simulink model "TorqueVect"  (Simulink 10.1)
settings: Solver=ode45  StartTime=0.0  StopTime=inf  RelTol=1e-3  EnableMultiTasking=on
PreLoadFcn:
  | run('Parameters\FSE_Parameters.m')
undefined symbols (not defined in the file): TC_Decr_Gas, TC_Derivative, TC_Incr_Gas, TC_On, TC_Relay_Off, TC_Relay_On, TV_On, TV_Override
libraries: CarMaker4SL x33, simulink x5, simulink_extras x4
(part 2 of 3)

== system TorqueVect/CarMaker/IPG Vehicle/CarAndTrailer/Forces/Tires ==
  note: The TireXX_Out signals will only be used if FileIdent is "CarMaker-Tire-CM4SL" in the tire parameter file!
      | An example parameter file can be found in Data/Tire/DT_CM4SL_UserTire.
  Sync_In : Inport
  TireFL_In : Inport  Port=2
  TireFR_In : Inport  Port=3
  TireRL_In : Inport  Port=4
  TireRR_In : Inport  Port=5
  Bus Creator{1..4} (4 alike) : BusCreator  Inputs=11
  Demux{1..3,8} (4 alike) : Demux  Outputs=7
      settings: DisplayOption=none
  TireFL : Subsystem
  TireFR : Subsystem
  TireRL : Subsystem
  TireRR : Subsystem
  TireFL_Out : Outport
  TireFR_Out : Outport  Port=2
  TireRL_Out : Outport  Port=3
  TireRR_Out : Outport  Port=4
  wires:
  Sync_In/1 -> TireRR/1(Sync_In), TireRL/1(Sync_In), TireFR/1(Sync_In), TireFL/1(Sync_In)
  Bus Creator4/1 -> TireRR_Out/1
  Bus Creator2/1 -> TireRL_Out/1
  Bus Creator1/1 -> TireFR_Out/1
  Demux3/5 -> TireRR/6(Rim_turnv)  "Tire_In Rim_turnv"
  Demux3/4 -> TireRR/5(Rim_rotv)  "Tire_In Rim_rotv"
  Demux3/1 -> TireRR/2(Load)  "Tire_In Load"
  Demux3/7 -> TireRR/8(muRoad)  "Tire_In mu"
  Demux3/6 -> TireRR/7(InclinAngle)  "Tire_In Camber"
  Demux3/2 -> TireRR/3(vxtrans)  "Tire_In vxtrans"
  Demux3/3 -> TireRR/4(vytrans)  "Tire_In vytrans"
  TireRR/11(AlignTrq) -> Bus Creator4/11  "Tire_Out AlignTrq"
  TireRR/10(RollResist) -> Bus Creator4/10  "Tire_Out RollResist"
  TireRR/9(OverturnTrq) -> Bus Creator4/9  "Tire_Out OverturnTrq"
  TireRR/8(LoadFrc) -> Bus Creator4/8  "Tire_Out LoadFrc"
  TireRR/7(SideFrc) -> Bus Creator4/7  "Tire_Out SideFrc"
  TireRR/6(LongFrc) -> Bus Creator4/6  "Tire_Out LongFrc"
  TireRR/5(vBelt) -> Bus Creator4/5  "Tire_Out vBelt"
  TireRR/4(rBelt_eff) -> Bus Creator4/4  "Tire_Out rBelt_eff"
  TireRR/3(TurnSlp) -> Bus Creator4/3  "Tire_Out TurnSlp"
  TireRR/1(Slp) -> Bus Creator4/1  "Tire_Out Slp"
  TireRR/2(Alpha) -> Bus Creator4/2  "Tire_Out Alpha"
  Demux2/5 -> TireRL/6(Rim_turnv)  "Tire_In Rim_turnv"
  Demux2/4 -> TireRL/5(Rim_rotv)  "Tire_In Rim_rotv"
  Demux2/1 -> TireRL/2(Load)  "Tire_In Load"
  Demux2/7 -> TireRL/8(muRoad)  "Tire_In mu"
  Demux2/6 -> TireRL/7(InclinAngle)  "Tire_In Camber"
  Demux2/2 -> TireRL/3(vxtrans)  "Tire_In vxtrans"
  Demux2/3 -> TireRL/4(vytrans)  "Tire_In vytrans"
  TireRL/11(AlignTrq) -> Bus Creator2/11  "Tire_Out AlignTrq"
  TireRL/10(RollResist) -> Bus Creator2/10  "Tire_Out RollResist"
  TireRL/9(OverturnTrq) -> Bus Creator2/9  "Tire_Out OverturnTrq"
  TireRL/8(LoadFrc) -> Bus Creator2/8  "Tire_Out LoadFrc"
  TireRL/7(SideFrc) -> Bus Creator2/7  "Tire_Out SideFrc"
  TireRL/6(LongFrc) -> Bus Creator2/6  "Tire_Out LongFrc"
  TireRL/5(vBelt) -> Bus Creator2/5  "Tire_Out vBelt"
  TireRL/4(rBelt_eff) -> Bus Creator2/4  "Tire_Out rBelt_eff"
  TireRL/3(TurnSlp) -> Bus Creator2/3  "Tire_Out TurnSlp"
  TireRL/1(Slp) -> Bus Creator2/1  "Tire_Out Slp"
  TireRL/2(Alpha) -> Bus Creator2/2  "Tire_Out Alpha"
  Demux1/5 -> TireFR/6(Rim_turnv)  "Tire_In Rim_turnv"
  Demux1/4 -> TireFR/5(Rim_rotv)  "Tire_In Rim_rotv"
  Demux1/1 -> TireFR/2(Load)  "Tire_In Load"
  Demux1/7 -> TireFR/8(muRoad)  "Tire_In mu"
  Demux1/6 -> TireFR/7(InclinAngle)  "Tire_In Camber"
  Demux1/2 -> TireFR/3(vxtrans)  "Tire_In vxtrans"
  Demux1/3 -> TireFR/4(vytrans)  "Tire_In vytrans"
  TireFR/11(AlignTrq) -> Bus Creator1/11  "Tire_Out AlignTrq"
  TireFR/10(RollResist) -> Bus Creator1/10  "Tire_Out RollResist"
  TireFR/9(OverturnTrq) -> Bus Creator1/9  "Tire_Out OverturnTrq"
  TireFR/8(LoadFrc) -> Bus Creator1/8  "Tire_Out LoadFrc"
  TireFR/7(SideFrc) -> Bus Creator1/7  "Tire_Out SideFrc"
  TireFR/6(LongFrc) -> Bus Creator1/6  "Tire_Out LongFrc"
  TireFR/5(vBelt) -> Bus Creator1/5  "Tire_Out vBelt"
  TireFR/4(rBelt_eff) -> Bus Creator1/4  "Tire_Out rBelt_eff"
  TireFR/3(TurnSlp) -> Bus Creator1/3  "Tire_Out TurnSlp"
  TireFR/1(Slp) -> Bus Creator1/1  "Tire_Out Slp"
  TireFR/2(Alpha) -> Bus Creator1/2  "Tire_Out Alpha"
  Demux8/5 -> TireFL/6(Rim_turnv)  "Tire_In Rim_turnv"
  Demux8/4 -> TireFL/5(Rim_rotv)  "Tire_In Rim_rotv"
  TireFL_In/1 -> Demux8/1
  Demux8/1 -> TireFL/2(Load)  "Tire_In Load"
  Demux8/7 -> TireFL/8(muRoad)  "Tire_In mu"
  Demux8/6 -> TireFL/7(InclinAngle)  "Tire_In Camber"
  Demux8/2 -> TireFL/3(vxtrans)  "Tire_In vxtrans"
  Demux8/3 -> TireFL/4(vytrans)  "Tire_In vytrans"
  TireFL/11(AlignTrq) -> Bus Creator3/11  "Tire_Out AlignTrq"
  TireFL/10(RollResist) -> Bus Creator3/10  "Tire_Out RollResist"
  TireFL/9(OverturnTrq) -> Bus Creator3/9  "Tire_Out OverturnTrq"
  TireFL/8(LoadFrc) -> Bus Creator3/8  "Tire_Out LoadFrc"
  TireFL/7(SideFrc) -> Bus Creator3/7  "Tire_Out SideFrc"
  TireFL/6(LongFrc) -> Bus Creator3/6  "Tire_Out LongFrc"
  TireFL/5(vBelt) -> Bus Creator3/5  "Tire_Out vBelt"
  TireFL/4(rBelt_eff) -> Bus Creator3/4  "Tire_Out rBelt_eff"
  TireFL/3(TurnSlp) -> Bus Creator3/3  "Tire_Out TurnSlp"
  TireFL/1(Slp) -> Bus Creator3/1  "Tire_Out Slp"
  TireFL/2(Alpha) -> Bus Creator3/2  "Tire_Out Alpha"
  Bus Creator3/1 -> TireFL_Out/1
  TireFR_In/1 -> Demux1/1
  TireRL_In/1 -> Demux2/1
  TireRR_In/1 -> Demux3/1

== system TorqueVect/CarMaker/IPG Vehicle/CarAndTrailer/Forces/Vehicle Forces ==
  Sync_In : Inport
  Bus Creator1 : BusCreator  Inputs=12
  Bus Creator8 : BusCreator  Inputs=16
  BusCreator1 : BusCreator  Inputs=4
  BusCreator2 : BusCreator  Inputs=9
  Demux : Demux  Outputs=16
      settings: DisplayOption=none
  Demux1 : Demux  Outputs=12
      settings: DisplayOption=none
  Demux2 : Demux  Outputs=13
      settings: DisplayOption=none
  Forces : S-Function  FunctionName=CM_Sfun  Parameters='Forces'  SFunctionDeploymentMode=off  EnableBusSupport=off
  Terminator : Terminator
  Sync_Out : Outport
  Car.Virtual : Outport  Port=2
  Car.Aero : Outport  Port=3
  Car.Load : Outport  Port=4
  wires:
  BusCreator1/1 -> Terminator/1  "Aero IF (in)"
  Demux2/13 -> BusCreator2/9  "car Aero Trq_1 z"
  Demux2/12 -> BusCreator2/8  "car Aero Trq_1 y"
  Demux2/11 -> BusCreator2/7  "car Aero Trq_1 x"
  Demux2/10 -> BusCreator2/6  "car Aero Frc_1 z"
  Demux2/9 -> BusCreator2/5  "car Aero Frc_1 y"
  Demux2/8 -> BusCreator2/4  "car Aero Frc_1 x"
  Demux2/7 -> BusCreator2/3  "car Aero PoA_1 z"
  Demux2/6 -> BusCreator2/2  "car Aero PoA_1 y"
  Demux2/5 -> BusCreator2/1  "car Aero PoA_1 x"
  Demux2/4 -> BusCreator1/4  "car Aero tau_1"
  Demux2/3 -> BusCreator1/3  "car Aero ApproachVel_1 z"
  Demux2/2 -> BusCreator1/2  "car Aero ApproachVel_1 y"
  Demux2/1 -> BusCreator1/1  "car Aero ApproachVel_1 x"
  Demux/16 -> Bus Creator8/16  "Car Load_3 tz"
  Demux/15 -> Bus Creator8/15  "Car Load_3 ty"
  Demux/14 -> Bus Creator8/14  "Car Load_3 tx"
  Demux/13 -> Bus Creator8/13  "Car Load_3 mass"
  Demux1/12 -> Bus Creator1/12  "Car Virtual Trq_0 z"
  Demux1/11 -> Bus Creator1/11  "Car Virtual Trq_0 y"
  Demux1/10 -> Bus Creator1/10  "Car Virtual Trq_0 x"
  Demux1/9 -> Bus Creator1/9  "Car Virtual Trq_1 z"
  Demux1/8 -> Bus Creator1/8  "Car Virtual Trq_1 y"
  Demux1/7 -> Bus Creator1/7  "Car Virtual Trq_1 x"
  Demux1/6 -> Bus Creator1/6  "Car Virtual Frc_0 z"
  Demux1/5 -> Bus Creator1/5  "Car Virtual Frc_0 y"
  Demux1/4 -> Bus Creator1/4  "Car Virtual Frc_0 x"
  Sync_In/1 -> Forces/1
  Forces/1 -> Sync_Out/1
  BusCreator2/1 -> Car.Aero/1
  Demux1/1 -> Bus Creator1/1  "Car Virtual Frc_1 x"
  Demux1/2 -> Bus Creator1/2  "Car Virtual Frc_1 y"
  Demux1/3 -> Bus Creator1/3  "Car Virtual Frc_1 z"
  Forces/3 -> Demux2/1
  Forces/2 -> Demux1/1
  Bus Creator1/1 -> Car.Virtual/1
  Bus Creator8/1 -> Car.Load/1
  Demux/1 -> Bus Creator8/1  "Car Load_0 mass"
  Demux/2 -> Bus Creator8/2  "Car Load_0 tx"
  Demux/3 -> Bus Creator8/3  "Car Load_0 ty"
  Demux/4 -> Bus Creator8/4  "Car Load_0 tz"
  Demux/5 -> Bus Creator8/5  "Car Load_1 mass"
  Demux/6 -> Bus Creator8/6  "Car Load_1 tx"
  Demux/7 -> Bus Creator8/7  "Car Load_1 ty"
  Demux/8 -> Bus Creator8/8  "Car Load_1 tz"
  Demux/9 -> Bus Creator8/9  "Car Load_2 mass"
  Demux/10 -> Bus Creator8/10  "Car Load_2 tx"
  Demux/11 -> Bus Creator8/11  "Car Load_2 ty"
  Demux/12 -> Bus Creator8/12  "Car Load_2 tz"
  Forces/4 -> Demux/1

== system TorqueVect/CarMaker/IPG Vehicle/CarAndTrailer/Trailer/CreateBus Car.Hitch.FrcTrq ==
  In1 : Inport
  Bus Creator7 : BusCreator  Inputs=6
  Demux7 : Demux  Outputs=6
      settings: DisplayOption=none
  Out1 : Outport
  wires:
  In1/1 -> Demux7/1
  Bus Creator7/1 -> Out1/1
  Demux7/6 -> Bus Creator7/6  "Car Hitch Trq2Car z"
  Demux7/5 -> Bus Creator7/5  "Car Hitch Trq2Car y"
  Demux7/4 -> Bus Creator7/4  "Car Hitch Trq2Car x"
  Demux7/3 -> Bus Creator7/3  "Car Hitch Frc2Car z"
  Demux7/2 -> Bus Creator7/2  "Car Hitch Frc2Car y"
  Demux7/1 -> Bus Creator7/1  "Car Hitch Frc2Car x"

== system TorqueVect/CarMaker/IPG Vehicle/CarAndTrailer/Trailer/CreateBus Vhcl.Motion ==
  In1 : Inport
  BusCreator : BusCreator  Inputs=15
  Demux : Demux  Outputs=15
      settings: DisplayOption=none
  Out1 : Outport
  wires:
  Demux/15 -> BusCreator/15  "Vhcl YawAcc"
  Demux/14 -> BusCreator/14  "Vhcl YawVel"
  Demux/13 -> BusCreator/13  "Vhcl Yaw"
  Demux/12 -> BusCreator/12  "Vhcl PitchAcc"
  Demux/11 -> BusCreator/11  "Vhcl PitchVel"
  Demux/10 -> BusCreator/10  "Vhcl Pitch"
  Demux/9 -> BusCreator/9  "Vhcl RollAcc"
  Demux/8 -> BusCreator/8  "Vhcl RollVel"
  Demux/7 -> BusCreator/7  "Vhcl Roll"
  Demux/6 -> BusCreator/6  "Vhcl Hitch_Pos z"
  Demux/5 -> BusCreator/5  "Vhcl Hitch_Pos y"
  Demux/4 -> BusCreator/4  "Vhcl Hitch_Pos x"
  Demux/3 -> BusCreator/3  "Vhcl sRoad"
  Demux/2 -> BusCreator/2  "Vhcl Distance"
  Demux/1 -> BusCreator/1  "Vhcl v"
  In1/1 -> Demux/1
  BusCreator/1 -> Out1/1

== system TorqueVect/CarMaker/IPG Vehicle/CarAndTrailer/Trailer/CreateBus Vhcl.PoI ==
  In1 : Inport
  Bus Creator3 : BusCreator  Inputs=18
  Demux3 : Demux  Outputs=18
      settings: DisplayOption=none
  Out1 : Outport
  wires:
  Demux3/18 -> Bus Creator3/18  "Vhcl PoI_GCS Elev"
  Demux3/17 -> Bus Creator3/17  "Vhcl PoI_GCS Lat"
  Demux3/16 -> Bus Creator3/16  "Vhcl PoI_GCS Long"
  Demux3/15 -> Bus Creator3/15  "Vhcl PoI_Acc_1 z"
  Demux3/14 -> Bus Creator3/14  "Vhcl PoI_Acc_1 y"
  Demux3/13 -> Bus Creator3/13  "Vhcl PoI_Acc_1 x"
  Demux3/12 -> Bus Creator3/12  "Vhcl PoI_Vel_1 z"
  Demux3/11 -> Bus Creator3/11  "Vhcl PoI_Vel_1 y"
  Demux3/10 -> Bus Creator3/10  "Vhcl PoI_Vel_1 x"
  Demux3/9 -> Bus Creator3/9  "Vhcl PoI_Acc z"
  Demux3/8 -> Bus Creator3/8  "Vhcl PoI_Acc y"
  Demux3/7 -> Bus Creator3/7  "Vhcl PoI_Acc x"
  Demux3/6 -> Bus Creator3/6  "Vhcl PoI_Vel z"
  Demux3/5 -> Bus Creator3/5  "Vhcl PoI_Vel y"
  Demux3/4 -> Bus Creator3/4  "Vhcl PoI_Vel x"
  Demux3/3 -> Bus Creator3/3  "Vhcl PoI_Pos z"
  Demux3/2 -> Bus Creator3/2  "Vhcl PoI_Pos y"
  In1/1 -> Demux3/1
  Bus Creator3/1 -> Out1/1
  Demux3/1 -> Bus Creator3/1  "Vhcl PoI_Pos x"

== system TorqueVect/CarMaker/IPG Vehicle/CarAndTrailer/Trailer/CreateBus Vhcl.Steering ==
  In1 : Inport
  Bus Creator3 : BusCreator  Inputs=4
  Demux : Demux
      settings: DisplayOption=none
  Out1 : Outport
  wires:
  Bus Creator3/1 -> Out1/1
  Demux/1 -> Bus Creator3/1  "Vhcl Steering Ang"
  Demux/3 -> Bus Creator3/3  "Vhcl Steering AngAcc"
  Demux/2 -> Bus Creator3/2  "Vhcl Steering AngVel"
  Demux/4 -> Bus Creator3/4  "Vhcl Steering Trq"
  In1/1 -> Demux/1

== system TorqueVect/CarMaker/IPG Vehicle/CarAndTrailer/Trailer/CreateBus Vhcl.Wheel.FL ==
  In1 : Inport
  Bus Creator3 : BusCreator  Inputs=14
  Demux3 : Demux  Outputs=14
      settings: DisplayOption=none
  Out1 : Outport
  wires:
  Demux3/14 -> Bus Creator3/14  "Vhcl Wheel FL Trq_WhlBearing"
  Demux3/13 -> Bus Creator3/13  "Vhcl Wheel FL Trq_T2W"
  Demux3/12 -> Bus Creator3/12  "Vhcl Wheel FL SideSlip"
  Demux3/11 -> Bus Creator3/11  "Vhcl Wheel FL LongSlip"
  Demux3/10 -> Bus Creator3/10  "Vhcl Wheel FL vBelt"
  Demux3/9 -> Bus Creator3/9  "Vhcl Wheel FL Fz"
  Demux3/8 -> Bus Creator3/8  "Vhcl Wheel FL Fy"
  Demux3/7 -> Bus Creator3/7  "Vhcl Wheel FL Fx"
  Demux3/6 -> Bus Creator3/6  "Vhcl Wheel FL r_zxy z"
  Demux3/5 -> Bus Creator3/5  "Vhcl Wheel FL r_zxy y"
  Demux3/4 -> Bus Creator3/4  "Vhcl Wheel FL r_zxy x"
  Demux3/3 -> Bus Creator3/3  "Vhcl Wheel FL t z"
  Demux3/2 -> Bus Creator3/2  "Vhcl Wheel FL t y"
  In1/1 -> Demux3/1
  Bus Creator3/1 -> Out1/1
  Demux3/1 -> Bus Creator3/1  "Vhcl Wheel FL t x"

== system TorqueVect/CarMaker/IPG Vehicle/CarAndTrailer/Trailer/CreateBus Vhcl.Wheel.FR ==
  In1 : Inport
  Bus Creator3 : BusCreator  Inputs=14
  Demux3 : Demux  Outputs=14
      settings: DisplayOption=none
  Out1 : Outport
  wires:
  Demux3/14 -> Bus Creator3/14  "Vhcl Wheel FR Trq_WhlBearing"
  Demux3/13 -> Bus Creator3/13  "Vhcl Wheel FR Trq_T2W"
  Demux3/12 -> Bus Creator3/12  "Vhcl Wheel FR SideSlip"
  Demux3/11 -> Bus Creator3/11  "Vhcl Wheel FR LongSlip"
  Demux3/10 -> Bus Creator3/10  "Vhcl Wheel FR vBelt"
  Demux3/9 -> Bus Creator3/9  "Vhcl Wheel FR Fz"
  Demux3/8 -> Bus Creator3/8  "Vhcl Wheel FR Fy"
  Demux3/7 -> Bus Creator3/7  "Vhcl Wheel FR Fx"
  Demux3/6 -> Bus Creator3/6  "Vhcl Wheel FR r_zxy z"
  Demux3/5 -> Bus Creator3/5  "Vhcl Wheel FR r_zxy y"
  Demux3/4 -> Bus Creator3/4  "Vhcl Wheel FR r_zxy x"
  Demux3/3 -> Bus Creator3/3  "Vhcl Wheel FR t z"
  Demux3/2 -> Bus Creator3/2  "Vhcl Wheel FR t y"
  In1/1 -> Demux3/1
  Bus Creator3/1 -> Out1/1
  Demux3/1 -> Bus Creator3/1  "Vhcl Wheel FR t x"

== system TorqueVect/CarMaker/IPG Vehicle/CarAndTrailer/Trailer/CreateBus Vhcl.Wheel.RL ==
  In1 : Inport
  Bus Creator3 : BusCreator  Inputs=14
  Demux3 : Demux  Outputs=14
      settings: DisplayOption=none
  Out1 : Outport
  wires:
  Demux3/14 -> Bus Creator3/14  "Vhcl Wheel RL Trq_WhlBearing"
  Demux3/13 -> Bus Creator3/13  "Vhcl Wheel RL Trq_T2W"
  Demux3/12 -> Bus Creator3/12  "Vhcl Wheel RL SideSlip"
  Demux3/11 -> Bus Creator3/11  "Vhcl Wheel RL LongSlip"
  Demux3/10 -> Bus Creator3/10  "Vhcl Wheel RL vBelt"
  Demux3/9 -> Bus Creator3/9  "Vhcl Wheel RL Fz"
  Demux3/8 -> Bus Creator3/8  "Vhcl Wheel RL Fy"
  Demux3/7 -> Bus Creator3/7  "Vhcl Wheel RL Fx"
  Demux3/6 -> Bus Creator3/6  "Vhcl Wheel RL r_zxy z"
  Demux3/5 -> Bus Creator3/5  "Vhcl Wheel RL r_zxy y"
  Demux3/4 -> Bus Creator3/4  "Vhcl Wheel RL r_zxy x"
  Demux3/3 -> Bus Creator3/3  "Vhcl Wheel RL t z"
  Demux3/2 -> Bus Creator3/2  "Vhcl Wheel RL t y"
  In1/1 -> Demux3/1
  Bus Creator3/1 -> Out1/1
  Demux3/1 -> Bus Creator3/1  "Vhcl Wheel RL t x"

== system TorqueVect/CarMaker/IPG Vehicle/CarAndTrailer/Trailer/CreateBus Vhcl.Wheel.RR ==
  In1 : Inport
  Bus Creator3 : BusCreator  Inputs=14
  Demux3 : Demux  Outputs=14
      settings: DisplayOption=none
  Out1 : Outport
  wires:
  Demux3/14 -> Bus Creator3/14  "Vhcl Wheel RR Trq_WhlBearing"
  Demux3/13 -> Bus Creator3/13  "Vhcl Wheel RR Trq_T2W"
  Demux3/12 -> Bus Creator3/12  "Vhcl Wheel RR SideSlip"
  Demux3/11 -> Bus Creator3/11  "Vhcl Wheel RR LongSlip"
  Demux3/10 -> Bus Creator3/10  "Vhcl Wheel RR vBelt"
  Demux3/9 -> Bus Creator3/9  "Vhcl Wheel RR Fz"
  Demux3/8 -> Bus Creator3/8  "Vhcl Wheel RR Fy"
  Demux3/7 -> Bus Creator3/7  "Vhcl Wheel RR Fx"
  Demux3/6 -> Bus Creator3/6  "Vhcl Wheel RR r_zxy z"
  Demux3/5 -> Bus Creator3/5  "Vhcl Wheel RR r_zxy y"
  Demux3/4 -> Bus Creator3/4  "Vhcl Wheel RR r_zxy x"
  Demux3/3 -> Bus Creator3/3  "Vhcl Wheel RR t z"
  Demux3/2 -> Bus Creator3/2  "Vhcl Wheel RR t y"
  In1/1 -> Demux3/1
  Bus Creator3/1 -> Out1/1
  Demux3/1 -> Bus Creator3/1  "Vhcl Wheel RR t x"

== system TorqueVect/CarMaker/IPG Vehicle/PowerTrain/PTControl Example/CreateBus PTC ClutchOut ==
  In : Inport
  BusCreator : BusCreator  Inputs=3
  Demux : Demux  Outputs=3
      settings: DisplayOption=none
  Out : Outport  VectorParamsAs1DForOutWhenUnconnected=off
  wires:
  In/1 -> Demux/1
  BusCreator/1 -> Out/1
  Demux/1 -> BusCreator/1  "PTC ClutchOut Pos"
  Demux/2 -> BusCreator/2  "PTC ClutchOut rotv_out_trg"
  Demux/3 -> BusCreator/3  "PTC ClutchOut Trq_out_trg"

== system TorqueVect/CarMaker/IPG Vehicle/PowerTrain/PTControl Example/CreateBus PTC EngineOut ==
  In : Inport
  BusCreator : BusCreator  Inputs=5
  Demux : Demux  Outputs=5
      settings: DisplayOption=none
  Out : Outport  VectorParamsAs1DForOutWhenUnconnected=off
  wires:
  In/1 -> Demux/1
  BusCreator/1 -> Out/1
  Demux/1 -> BusCreator/1  "PTC EngineOut set_ISC"
  Demux/2 -> BusCreator/2  "PTC EngineOut FuelCutOff"
  Demux/3 -> BusCreator/3  "PTC EngineOut Load"
  Demux/4 -> BusCreator/4  "PTC EngineOut Trq_trg"
  Demux/5 -> BusCreator/5  "PTC EngineOut rotv_trg"

== system TorqueVect/CarMaker/IPG Vehicle/PowerTrain/PTControl Example/CreateBus PTC GearBoxM_Out0 ==
  In : Inport
  BusCreator : BusCreator  Inputs=12
  Demux : Demux  Outputs=12
      settings: DisplayOption=none
  Out : Outport  VectorParamsAs1DForOutWhenUnconnected=off
  wires:
  In/1 -> Demux/1
  BusCreator/1 -> Out/1
  Demux/1 -> BusCreator/1  "PTC GearBoxM_Out0 GearNoTrg"
  Demux/2 -> BusCreator/2  "PTC GearBoxM_Out0 GearNoTrg_dis"
  Demux/3 -> BusCreator/3  "PTC GearBoxM_Out0 set_ParkBrake"
  Demux/4 -> BusCreator/4  "PTC GearBoxM_Out0 i_trg"
  Demux/5 -> BusCreator/5  "PTC GearBoxM_Out0 rotv_in_trg"
  Demux/6 -> BusCreator/6  "PTC GearBoxM_Out0 Trq_out_trg"
  Demux/7 -> BusCreator/7  "PTC GearBoxM_Out0 Clutch Pos"
  Demux/8 -> BusCreator/8  "PTC GearBoxM_Out0 Clutch rotv_out_trg"
  Demux/9 -> BusCreator/9  "PTC GearBoxM_Out0 Clutch Trq_out_trg"
  Demux/10 -> BusCreator/10  "PTC GearBoxM_Out0 Clutch_dis Pos"
  Demux/11 -> BusCreator/11  "PTC GearBoxM_Out0 Clutch_dis rotv_out_trg"
  Demux/12 -> BusCreator/12  "PTC GearBoxM_Out0 Clutch_dis Trq_out_trg"

== system TorqueVect/CarMaker/IPG Vehicle/PowerTrain/PTControl Example/CreateBus PTC GearBoxM_Out1 ==
  In : Inport
  BusCreator : BusCreator  Inputs=12
  Demux : Demux  Outputs=12
      settings: DisplayOption=none
  Out : Outport  VectorParamsAs1DForOutWhenUnconnected=off
  wires:
  In/1 -> Demux/1
  BusCreator/1 -> Out/1
  Demux/1 -> BusCreator/1  "PTC GearBoxM_Out1 GearNoTrg"
  Demux/2 -> BusCreator/2  "PTC GearBoxM_Out1 GearNoTrg_dis"
  Demux/3 -> BusCreator/3  "PTC GearBoxM_Out1 set_ParkBrake"
  Demux/4 -> BusCreator/4  "PTC GearBoxM_Out1 i_trg"
  Demux/5 -> BusCreator/5  "PTC GearBoxM_Out1 rotv_in_trg"
  Demux/6 -> BusCreator/6  "PTC GearBoxM_Out1 Trq_out_trg"
  Demux/7 -> BusCreator/7  "PTC GearBoxM_Out1 Clutch Pos"
  Demux/8 -> BusCreator/8  "PTC GearBoxM_Out1 Clutch rotv_out_trg"
  Demux/9 -> BusCreator/9  "PTC GearBoxM_Out1 Clutch Trq_out_trg"
  Demux/10 -> BusCreator/10  "PTC GearBoxM_Out1 Clutch_dis Pos"
  Demux/11 -> BusCreator/11  "PTC GearBoxM_Out1 Clutch_dis rotv_out_trg"
  Demux/12 -> BusCreator/12  "PTC GearBoxM_Out1 Clutch_dis Trq_out_trg"

== system TorqueVect/CarMaker/IPG Vehicle/PowerTrain/PTControl Example/CreateBus PTC GearBoxM_Out2 ==
  In : Inport
  BusCreator : BusCreator  Inputs=12
  Demux : Demux  Outputs=12
      settings: DisplayOption=none
  Out : Outport  VectorParamsAs1DForOutWhenUnconnected=off
  wires:
  In/1 -> Demux/1
  BusCreator/1 -> Out/1
  Demux/1 -> BusCreator/1  "PTC GearBoxM_Out2 GearNoTrg"
  Demux/2 -> BusCreator/2  "PTC GearBoxM_Out2 GearNoTrg_dis"
  Demux/3 -> BusCreator/3  "PTC GearBoxM_Out2 set_ParkBrake"
  Demux/4 -> BusCreator/4  "PTC GearBoxM_Out2 i_trg"
  Demux/5 -> BusCreator/5  "PTC GearBoxM_Out2 rotv_in_trg"
  Demux/6 -> BusCreator/6  "PTC GearBoxM_Out2 Trq_out_trg"
  Demux/7 -> BusCreator/7  "PTC GearBoxM_Out2 Clutch Pos"
  Demux/8 -> BusCreator/8  "PTC GearBoxM_Out2 Clutch rotv_out_trg"
  Demux/9 -> BusCreator/9  "PTC GearBoxM_Out2 Clutch Trq_out_trg"
  Demux/10 -> BusCreator/10  "PTC GearBoxM_Out2 Clutch_dis Pos"
  Demux/11 -> BusCreator/11  "PTC GearBoxM_Out2 Clutch_dis rotv_out_trg"
  Demux/12 -> BusCreator/12  "PTC GearBoxM_Out2 Clutch_dis Trq_out_trg"

== system TorqueVect/CarMaker/IPG Vehicle/PowerTrain/PTControl Example/CreateBus PTC GearBoxM_Out3 ==
  In : Inport
  BusCreator : BusCreator  Inputs=12
  Demux : Demux  Outputs=12
      settings: DisplayOption=none
  Out : Outport  VectorParamsAs1DForOutWhenUnconnected=off
  wires:
  In/1 -> Demux/1
  BusCreator/1 -> Out/1
  Demux/1 -> BusCreator/1  "PTC GearBoxM_Out3 GearNoTrg"
  Demux/2 -> BusCreator/2  "PTC GearBoxM_Out3 GearNoTrg_dis"
  Demux/3 -> BusCreator/3  "PTC GearBoxM_Out3 set_ParkBrake"
  Demux/4 -> BusCreator/4  "PTC GearBoxM_Out3 i_trg"
  Demux/5 -> BusCreator/5  "PTC GearBoxM_Out3 rotv_in_trg"
  Demux/6 -> BusCreator/6  "PTC GearBoxM_Out3 Trq_out_trg"
  Demux/7 -> BusCreator/7  "PTC GearBoxM_Out3 Clutch Pos"
  Demux/8 -> BusCreator/8  "PTC GearBoxM_Out3 Clutch rotv_out_trg"
  Demux/9 -> BusCreator/9  "PTC GearBoxM_Out3 Clutch Trq_out_trg"
  Demux/10 -> BusCreator/10  "PTC GearBoxM_Out3 Clutch_dis Pos"
  Demux/11 -> BusCreator/11  "PTC GearBoxM_Out3 Clutch_dis rotv_out_trg"
  Demux/12 -> BusCreator/12  "PTC GearBoxM_Out3 Clutch_dis Trq_out_trg"

== system TorqueVect/CarMaker/IPG Vehicle/PowerTrain/PTControl Example/CreateBus PTC GearBoxOut ==
  In : Inport
  BusCreator : BusCreator  Inputs=12
  Demux : Demux  Outputs=12
      settings: DisplayOption=none
  Out : Outport  VectorParamsAs1DForOutWhenUnconnected=off
  wires:
  In/1 -> Demux/1
  BusCreator/1 -> Out/1
  Demux/1 -> BusCreator/1  "PTC GearBoxOut GearNoTrg"
  Demux/2 -> BusCreator/2  "PTC GearBoxOut GearNoTrg_dis"
  Demux/3 -> BusCreator/3  "PTC GearBoxOut set_ParkBrake"
  Demux/4 -> BusCreator/4  "PTC GearBoxOut i_trg"
  Demux/5 -> BusCreator/5  "PTC GearBoxOut rotv_in_trg"
  Demux/6 -> BusCreator/6  "PTC GearBoxOut Trq_out_trg"
  Demux/7 -> BusCreator/7  "PTC GearBoxOut Clutch Pos"
  Demux/8 -> BusCreator/8  "PTC GearBoxOut Clutch rotv_out_trg"
  Demux/9 -> BusCreator/9  "PTC GearBoxOut Clutch Trq_out_trg"
  Demux/10 -> BusCreator/10  "PTC GearBoxOut Clutch_dis Pos"
  Demux/11 -> BusCreator/11  "PTC GearBoxOut Clutch_dis rotv_out_trg"
  Demux/12 -> BusCreator/12  "PTC GearBoxOut Clutch_dis Trq_out_trg"

== system TorqueVect/CarMaker/IPG Vehicle/PowerTrain/PTControl Example/CreateBus PTC ISGOut ==
  In : Inport
  BusCreator : BusCreator  Inputs=3
  Demux : Demux  Outputs=3
      settings: DisplayOption=none
  Out : Outport  VectorParamsAs1DForOutWhenUnconnected=off
  wires:
  In/1 -> Demux/1
  BusCreator/1 -> Out/1
  Demux/1 -> BusCreator/1  "PTC ISGOut Load"
  Demux/2 -> BusCreator/2  "PTC ISGOut Trq_trg"
  Demux/3 -> BusCreator/3  "PTC ISGOut rotv_trg"

== system TorqueVect/CarMaker/IPG Vehicle/PowerTrain/PTControl Example/CreateBus PTC MiscOut ==
  In : Inport
  BusCreator : BusCreator  Inputs=4
  Demux : Demux
      settings: DisplayOption=none
  Out : Outport  VectorParamsAs1DForOutWhenUnconnected=off
  wires:
  In/1 -> Demux/1
  BusCreator/1 -> Out/1
  Demux/1 -> BusCreator/1  "PTC_Out OperationState"
  Demux/2 -> BusCreator/2  "PTC_Out OperationError"
  Demux/3 -> BusCreator/3  "PTC_Out StrategyMode"
  Demux/4 -> BusCreator/4  "PTC_Out Ignition"

== system TorqueVect/CarMaker/IPG Vehicle/PowerTrain/PTControl Example/CreateBus PTC MotorOut0 ==
  In : Inport
  BusCreator : BusCreator  Inputs=3
  Demux : Demux  Outputs=3
      settings: DisplayOption=none
  Out : Outport  VectorParamsAs1DForOutWhenUnconnected=off
  wires:
  In/1 -> Demux/1
  BusCreator/1 -> Out/1
  Demux/1 -> BusCreator/1  "PTC MotorOut0 Load"
  Demux/2 -> BusCreator/2  "PTC MotorOut0 Trq_trg"
  Demux/3 -> BusCreator/3  "PTC MotorOut0 rotv_trg"

== system TorqueVect/CarMaker/IPG Vehicle/PowerTrain/PTControl Example/CreateBus PTC MotorOut1 ==
  In : Inport
  BusCreator : BusCreator  Inputs=3
  Demux : Demux  Outputs=3
      settings: DisplayOption=none
  Out : Outport  VectorParamsAs1DForOutWhenUnconnected=off
  wires:
  In/1 -> Demux/1
  BusCreator/1 -> Out/1
  Demux/1 -> BusCreator/1  "PTC MotorOut1 Load"
  Demux/2 -> BusCreator/2  "PTC MotorOut1 Trq_trg"
  Demux/3 -> BusCreator/3  "PTC MotorOut1 rotv_trg"

== system TorqueVect/CarMaker/IPG Vehicle/PowerTrain/PTControl Example/CreateBus PTC MotorOut2 ==
  In : Inport
  BusCreator : BusCreator  Inputs=3
  Demux : Demux  Outputs=3
      settings: DisplayOption=none
  Out : Outport  VectorParamsAs1DForOutWhenUnconnected=off
  wires:
  In/1 -> Demux/1
  BusCreator/1 -> Out/1
  Demux/1 -> BusCreator/1  "PTC MotorOut2 Load"
  Demux/2 -> BusCreator/2  "PTC MotorOut2 Trq_trg"
  Demux/3 -> BusCreator/3  "PTC MotorOut2 rotv_trg"

== system TorqueVect/CarMaker/IPG Vehicle/PowerTrain/PTControl Example/CreateBus PTC MotorOut3 ==
  In : Inport
  BusCreator : BusCreator  Inputs=3
  Demux : Demux  Outputs=3
      settings: DisplayOption=none
  Out : Outport  VectorParamsAs1DForOutWhenUnconnected=off
  wires:
  In/1 -> Demux/1
  BusCreator/1 -> Out/1
  Demux/1 -> BusCreator/1  "PTC MotorOut3 Load"
  Demux/2 -> BusCreator/2  "PTC MotorOut3 Trq_trg"
  Demux/3 -> BusCreator/3  "PTC MotorOut3 rotv_trg"

== system TorqueVect/CarMaker/IPG Vehicle/PowerTrain/PTControl Example/CreateBus PTC PwrSupplyOut ==
  In : Inport
  BusCreator : BusCreator  Inputs=1
  Demux : Demux  Outputs=1
      settings: DisplayOption=none
  Out : Outport  VectorParamsAs1DForOutWhenUnconnected=off
  wires:
  In/1 -> Demux/1
  BusCreator/1 -> Out/1
  Demux/1 -> BusCreator/1  "PTC PwrSupplyOut Pwr_HV1toLV_trg"

== system TorqueVect/CarMaker/IPG Vehicle/PowerTrain/PTControl Example/CreateBus PTC WheelOut ==
  In : Inport
  BusCreator : BusCreator  Inputs=8
  Demux : Demux  Outputs=8
      settings: DisplayOption=none
  Out : Outport  VectorParamsAs1DForOutWhenUnconnected=off
  wires:
  In/1 -> Demux/1
  BusCreator/1 -> Out/1
  Demux/1 -> BusCreator/1  "PTC WheelOut_FL Trq_BrakeReg"
  Demux/2 -> BusCreator/2  "PTC WheelOut_FL Trq_BrakeReg_max"
  Demux/3 -> BusCreator/3  "PTC WheelOut_FR Trq_BrakeReg"
  Demux/4 -> BusCreator/4  "PTC WheelOut_FR Trq_BrakeReg_max"
  Demux/5 -> BusCreator/5  "PTC WheelOut_RL Trq_BrakeReg"
  Demux/6 -> BusCreator/6  "PTC WheelOut_RL Trq_BrakeReg_max"
  Demux/7 -> BusCreator/7  "PTC WheelOut_RR Trq_BrakeReg"
  Demux/8 -> BusCreator/8  "PTC WheelOut_RR Trq_BrakeReg_max"

== system TorqueVect/CarMaker/IPG Vehicle/PowerTrain/PTControl Example/PTControl ==
  note: Minimalistic PTControl
      | example model
      | to be used with
      | FSE_TorqueVectoring
  VhclCtrl.PT : Inport
  Bus Selector : BusSelector  OutputSignals=VhclCtrl Gas
  PTC : Subsystem
  Torque Control 0 : Subsystem
  Torque Control 1 : Subsystem
  Torque Control 2 : Subsystem
  Torque Control 3 : Subsystem
  PTC MiscOut : Outport  VectorParamsAs1DForOutWhenUnconnected=off
  MotorOut0 : Outport  Port=2  VectorParamsAs1DForOutWhenUnconnected=off
  MotorOut1 : Outport  Port=3  VectorParamsAs1DForOutWhenUnconnected=off
  MotorOut2 : Outport  Port=4  VectorParamsAs1DForOutWhenUnconnected=off
  MotorOut3 : Outport  Port=5  VectorParamsAs1DForOutWhenUnconnected=off
  wires:
  Bus Selector/1 -> Torque Control 1/1(Gas), Torque Control 0/1(Gas), Torque Control 3/1(Gas), Torque Control 2/1(Gas)  "<VhclCtrl Gas>"
  Torque Control 3/1(MotorOut3) -> MotorOut3/1
  Torque Control 2/1(MotorOut2) -> MotorOut2/1
  Torque Control 1/1(MotorOut1) -> MotorOut1/1
  VhclCtrl.PT/1 -> Bus Selector/1
  Torque Control 0/1(MotorOut0) -> MotorOut0/1
  PTC/1(PTC MiscOut) -> PTC MiscOut/1

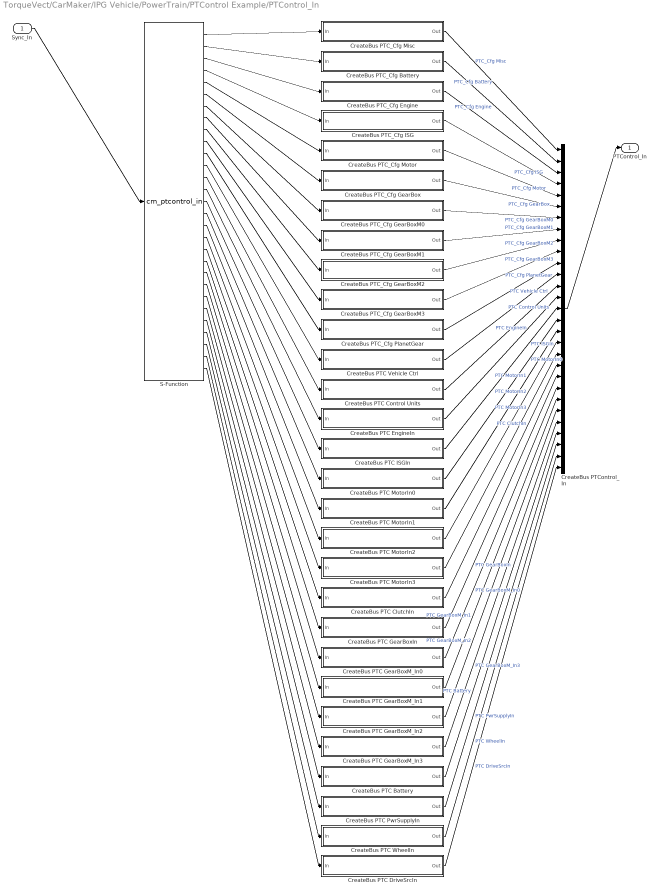
== system TorqueVect/CarMaker/IPG Vehicle/PowerTrain/PTControl Example/PTControl_In ==
  Sync_In : Inport
  CreateBus PTC Battery : Subsystem
  CreateBus PTC ClutchIn : Subsystem
  CreateBus PTC Control Units : Subsystem
  CreateBus PTC DriveSrcIn : Subsystem
  CreateBus PTC EngineIn : Subsystem
  CreateBus PTC GearBoxIn : Subsystem
  CreateBus PTC GearBoxM_In0 : Subsystem
  CreateBus PTC GearBoxM_In1 : Subsystem
  CreateBus PTC GearBoxM_In2 : Subsystem
  CreateBus PTC GearBoxM_In3 : Subsystem
  CreateBus PTC ISGIn : Subsystem
  CreateBus PTC MotorIn0 : Subsystem
  CreateBus PTC MotorIn1 : Subsystem
  CreateBus PTC MotorIn2 : Subsystem
  CreateBus PTC MotorIn3 : Subsystem
  CreateBus PTC PwrSupplyIn : Subsystem
  CreateBus PTC Vehicle Ctrl : Subsystem
  CreateBus PTC WheelIn : Subsystem
  CreateBus PTC_Cfg Battery : Subsystem
  CreateBus PTC_Cfg Engine : Subsystem
  CreateBus PTC_Cfg GearBox : Subsystem
  CreateBus PTC_Cfg GearBoxM0 : Subsystem
  CreateBus PTC_Cfg GearBoxM1 : Subsystem
  CreateBus PTC_Cfg GearBoxM2 : Subsystem
  CreateBus PTC_Cfg GearBoxM3 : Subsystem
  CreateBus PTC_Cfg ISG : Subsystem
  CreateBus PTC_Cfg Misc : Subsystem
  CreateBus PTC_Cfg Motor : Subsystem
  CreateBus PTC_Cfg PlanetGear : Subsystem
  CreateBus PTControl_In : BusCreator  Inputs=29
  S-Function : S-Function  FunctionName=cm_ptcontrol_in  SFunctionDeploymentMode=off  EnableBusSupport=off
  PTControl_In : Outport  VectorParamsAs1DForOutWhenUnconnected=off
  wires:
  Sync_In/1 -> S-Function/1
  CreateBus PTControl_In/1 -> PTControl_In/1
  S-Function/1 -> CreateBus PTC_Cfg Misc/1(In)
  CreateBus PTC_Cfg Misc/1(Out) -> CreateBus PTControl_In/1  "PTC_Cfg Misc"
  S-Function/2 -> CreateBus PTC_Cfg Battery/1(In)
  CreateBus PTC_Cfg Battery/1(Out) -> CreateBus PTControl_In/2  "PTC_Cfg Battery"
  S-Function/3 -> CreateBus PTC_Cfg Engine/1(In)
  CreateBus PTC_Cfg Engine/1(Out) -> CreateBus PTControl_In/3  "PTC_Cfg Engine"
  S-Function/4 -> CreateBus PTC_Cfg ISG/1(In)
  CreateBus PTC_Cfg ISG/1(Out) -> CreateBus PTControl_In/4  "PTC_Cfg ISG"
  S-Function/5 -> CreateBus PTC_Cfg Motor/1(In)
  CreateBus PTC_Cfg Motor/1(Out) -> CreateBus PTControl_In/5  "PTC_Cfg Motor"
  S-Function/6 -> CreateBus PTC_Cfg GearBox/1(In)
  CreateBus PTC_Cfg GearBox/1(Out) -> CreateBus PTControl_In/6  "PTC_Cfg GearBox"
  S-Function/7 -> CreateBus PTC_Cfg GearBoxM0/1(In)
  CreateBus PTC_Cfg GearBoxM0/1(Out) -> CreateBus PTControl_In/7  "PTC_Cfg GearBoxM0"
  S-Function/8 -> CreateBus PTC_Cfg GearBoxM1/1(In)
  CreateBus PTC_Cfg GearBoxM1/1(Out) -> CreateBus PTControl_In/8  "PTC_Cfg GearBoxM1"
  S-Function/9 -> CreateBus PTC_Cfg GearBoxM2/1(In)
  CreateBus PTC_Cfg GearBoxM2/1(Out) -> CreateBus PTControl_In/9  "PTC_Cfg GearBoxM2"
  S-Function/10 -> CreateBus PTC_Cfg GearBoxM3/1(In)
  CreateBus PTC_Cfg GearBoxM3/1(Out) -> CreateBus PTControl_In/10  "PTC_Cfg GearBoxM3"
  S-Function/11 -> CreateBus PTC_Cfg PlanetGear/1(In)
  CreateBus PTC_Cfg PlanetGear/1(Out) -> CreateBus PTControl_In/11  "PTC_Cfg PlanetGear"
  S-Function/12 -> CreateBus PTC Vehicle Ctrl/1(In)
  CreateBus PTC Vehicle Ctrl/1(Out) -> CreateBus PTControl_In/12  "PTC Vehicle Ctrl"
  S-Function/13 -> CreateBus PTC Control Units/1(In)
  CreateBus PTC Control Units/1(Out) -> CreateBus PTControl_In/13  "PTC Control Units"
  S-Function/14 -> CreateBus PTC EngineIn/1(In)
  CreateBus PTC EngineIn/1(Out) -> CreateBus PTControl_In/14  "PTC EngineIn"
  S-Function/15 -> CreateBus PTC ISGIn/1(In)
  CreateBus PTC ISGIn/1(Out) -> CreateBus PTControl_In/15  "PTC ISGIn"
  S-Function/16 -> CreateBus PTC MotorIn0/1(In)
  CreateBus PTC MotorIn0/1(Out) -> CreateBus PTControl_In/16  "PTC MotorIn0"
  S-Function/17 -> CreateBus PTC MotorIn1/1(In)
  CreateBus PTC MotorIn1/1(Out) -> CreateBus PTControl_In/17  "PTC MotorIn1"
  S-Function/18 -> CreateBus PTC MotorIn2/1(In)
  CreateBus PTC MotorIn2/1(Out) -> CreateBus PTControl_In/18  "PTC MotorIn2"
  S-Function/19 -> CreateBus PTC MotorIn3/1(In)
  CreateBus PTC MotorIn3/1(Out) -> CreateBus PTControl_In/19  "PTC MotorIn3"
  S-Function/20 -> CreateBus PTC ClutchIn/1(In)
  CreateBus PTC ClutchIn/1(Out) -> CreateBus PTControl_In/20  "PTC ClutchIn"
  S-Function/21 -> CreateBus PTC GearBoxIn/1(In)
  CreateBus PTC GearBoxIn/1(Out) -> CreateBus PTControl_In/21  "PTC GearBoxIn"
  S-Function/22 -> CreateBus PTC GearBoxM_In0/1(In)
  CreateBus PTC GearBoxM_In0/1(Out) -> CreateBus PTControl_In/22  "PTC GearBoxM_In0"
  S-Function/23 -> CreateBus PTC GearBoxM_In1/1(In)
  CreateBus PTC GearBoxM_In1/1(Out) -> CreateBus PTControl_In/23  "PTC GearBoxM_In1"
  S-Function/24 -> CreateBus PTC GearBoxM_In2/1(In)
  CreateBus PTC GearBoxM_In2/1(Out) -> CreateBus PTControl_In/24  "PTC GearBoxM_In2"
  S-Function/25 -> CreateBus PTC GearBoxM_In3/1(In)
  CreateBus PTC GearBoxM_In3/1(Out) -> CreateBus PTControl_In/25  "PTC GearBoxM_In3"
  S-Function/26 -> CreateBus PTC Battery/1(In)
  CreateBus PTC Battery/1(Out) -> CreateBus PTControl_In/26  "PTC Battery"
  S-Function/27 -> CreateBus PTC PwrSupplyIn/1(In)
  CreateBus PTC PwrSupplyIn/1(Out) -> CreateBus PTControl_In/27  "PTC PwrSupplyIn"
  S-Function/28 -> CreateBus PTC WheelIn/1(In)
  CreateBus PTC WheelIn/1(Out) -> CreateBus PTControl_In/28  "PTC WheelIn"
  S-Function/29 -> CreateBus PTC DriveSrcIn/1(In)
  CreateBus PTC DriveSrcIn/1(Out) -> CreateBus PTControl_In/29  "PTC DriveSrcIn"

== system TorqueVect/CarMaker/IPG Vehicle/PowerTrain/PTControl Example/PTControl_Out ==
  PTC MiscOut : Inport
  PTC EngineOut : Inport  Port=2
  PTC ISGOut : Inport  Port=3
  PTC MotorOut0 : Inport  Port=4
  PTC MotorOut1 : Inport  Port=5
  PTC MotorOut2 : Inport  Port=6
  PTC MotorOut3 : Inport  Port=7
  PTC ClutchOut : Inport  Port=8
  PTC GearBoxOut : Inport  Port=9
  PTC GearBoxM_Out0 : Inport  Port=10
  PTC GearBoxM_Out1 : Inport  Port=11
  PTC GearBoxM_Out2 : Inport  Port=12
  PTC GearBoxM_Out3 : Inport  Port=13
  PTC PwrSupplyOut : Inport  Port=14
  PTC WheelOut : Inport  Port=15
  PTControl_Out : S-Function  FunctionName=cm_ptcontrol_out  SFunctionDeploymentMode=off  EnableBusSupport=off
  wires:
  PTC MiscOut/1 -> PTControl_Out/1
  PTC EngineOut/1 -> PTControl_Out/2
  PTC ISGOut/1 -> PTControl_Out/3
  PTC MotorOut0/1 -> PTControl_Out/4
  PTC MotorOut1/1 -> PTControl_Out/5
  PTC MotorOut2/1 -> PTControl_Out/6
  PTC MotorOut3/1 -> PTControl_Out/7
  PTC ClutchOut/1 -> PTControl_Out/8
  PTC GearBoxOut/1 -> PTControl_Out/9
  PTC GearBoxM_Out0/1 -> PTControl_Out/10
  PTC GearBoxM_Out1/1 -> PTControl_Out/11
  PTC GearBoxM_Out2/1 -> PTControl_Out/12
  PTC GearBoxM_Out3/1 -> PTControl_Out/13
  PTC PwrSupplyOut/1 -> PTControl_Out/14
  PTC WheelOut/1 -> PTControl_Out/15

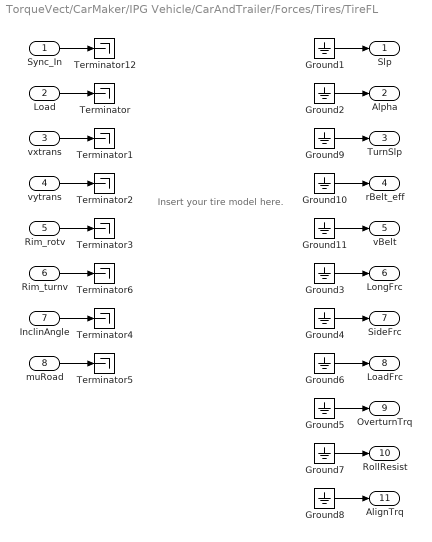
== system TorqueVect/CarMaker/IPG Vehicle/CarAndTrailer/Forces/Tires/TireFL ==
  note: Insert your tire model here.
  Sync_In : Inport
  Load : Inport  Port=2
  vxtrans : Inport  Port=3
  vytrans : Inport  Port=4
  Rim_rotv : Inport  Port=5
  Rim_turnv : Inport  Port=6
  InclinAngle : Inport  Port=7
  muRoad : Inport  Port=8
  Ground{1..11} (11 alike) : Ground
  Terminator{,1..6,12} (8 alike) : Terminator
  Slp : Outport
  Alpha : Outport  Port=2
  TurnSlp : Outport  Port=3
  rBelt_eff : Outport  Port=4
  vBelt : Outport  Port=5
  LongFrc : Outport  Port=6
  SideFrc : Outport  Port=7
  LoadFrc : Outport  Port=8
  OverturnTrq : Outport  Port=9
  RollResist : Outport  Port=10
  AlignTrq : Outport  Port=11
  wires:
  Ground11/1 -> vBelt/1
  Ground10/1 -> rBelt_eff/1
  Ground9/1 -> TurnSlp/1
  Rim_turnv/1 -> Terminator6/1
  Sync_In/1 -> Terminator12/1
  Ground2/1 -> Alpha/1
  Ground3/1 -> LongFrc/1
  Ground4/1 -> SideFrc/1
  Ground5/1 -> OverturnTrq/1
  vxtrans/1 -> Terminator1/1
  vytrans/1 -> Terminator2/1
  Rim_rotv/1 -> Terminator3/1
  InclinAngle/1 -> Terminator4/1
  muRoad/1 -> Terminator5/1
  Load/1 -> Terminator/1
  Ground1/1 -> Slp/1
  Ground6/1 -> LoadFrc/1
  Ground7/1 -> RollResist/1
  Ground8/1 -> AlignTrq/1

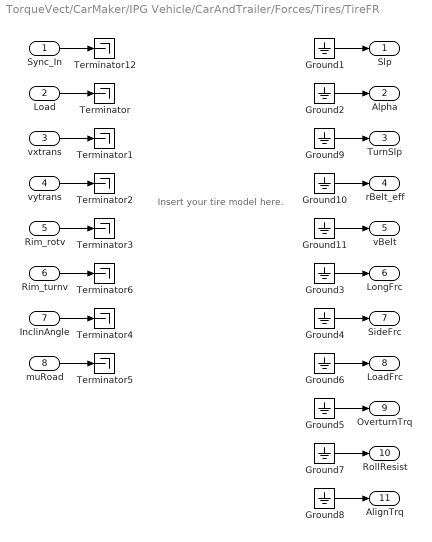
== system TorqueVect/CarMaker/IPG Vehicle/CarAndTrailer/Forces/Tires/TireFR ==
  note: Insert your tire model here.
  Sync_In : Inport
  Load : Inport  Port=2
  vxtrans : Inport  Port=3
  vytrans : Inport  Port=4
  Rim_rotv : Inport  Port=5
  Rim_turnv : Inport  Port=6
  InclinAngle : Inport  Port=7
  muRoad : Inport  Port=8
  Ground{1..11} (11 alike) : Ground
  Terminator{,1..6,12} (8 alike) : Terminator
  Slp : Outport
  Alpha : Outport  Port=2
  TurnSlp : Outport  Port=3
  rBelt_eff : Outport  Port=4
  vBelt : Outport  Port=5
  LongFrc : Outport  Port=6
  SideFrc : Outport  Port=7
  LoadFrc : Outport  Port=8
  OverturnTrq : Outport  Port=9
  RollResist : Outport  Port=10
  AlignTrq : Outport  Port=11
  wires:
  Ground11/1 -> vBelt/1
  Ground10/1 -> rBelt_eff/1
  Ground9/1 -> TurnSlp/1
  Rim_turnv/1 -> Terminator6/1
  Sync_In/1 -> Terminator12/1
  Ground2/1 -> Alpha/1
  Ground3/1 -> LongFrc/1
  Ground4/1 -> SideFrc/1
  Ground5/1 -> OverturnTrq/1
  vxtrans/1 -> Terminator1/1
  vytrans/1 -> Terminator2/1
  Rim_rotv/1 -> Terminator3/1
  InclinAngle/1 -> Terminator4/1
  muRoad/1 -> Terminator5/1
  Load/1 -> Terminator/1
  Ground1/1 -> Slp/1
  Ground6/1 -> LoadFrc/1
  Ground7/1 -> RollResist/1
  Ground8/1 -> AlignTrq/1

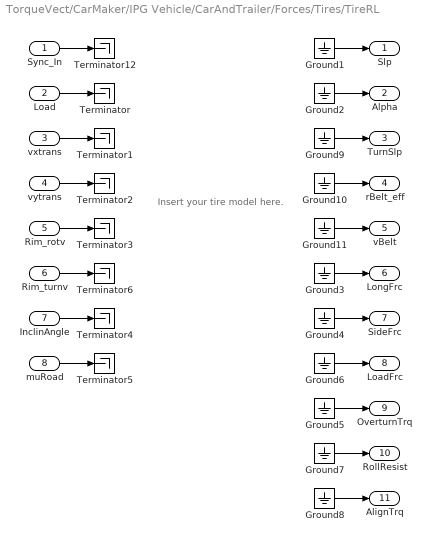
== system TorqueVect/CarMaker/IPG Vehicle/CarAndTrailer/Forces/Tires/TireRL ==
  note: Insert your tire model here.
  Sync_In : Inport
  Load : Inport  Port=2
  vxtrans : Inport  Port=3
  vytrans : Inport  Port=4
  Rim_rotv : Inport  Port=5
  Rim_turnv : Inport  Port=6
  InclinAngle : Inport  Port=7
  muRoad : Inport  Port=8
  Ground{1..11} (11 alike) : Ground
  Terminator{,1..6,12} (8 alike) : Terminator
  Slp : Outport
  Alpha : Outport  Port=2
  TurnSlp : Outport  Port=3
  rBelt_eff : Outport  Port=4
  vBelt : Outport  Port=5
  LongFrc : Outport  Port=6
  SideFrc : Outport  Port=7
  LoadFrc : Outport  Port=8
  OverturnTrq : Outport  Port=9
  RollResist : Outport  Port=10
  AlignTrq : Outport  Port=11
  wires:
  Ground11/1 -> vBelt/1
  Ground10/1 -> rBelt_eff/1
  Ground9/1 -> TurnSlp/1
  Rim_turnv/1 -> Terminator6/1
  Sync_In/1 -> Terminator12/1
  Ground2/1 -> Alpha/1
  Ground3/1 -> LongFrc/1
  Ground4/1 -> SideFrc/1
  Ground5/1 -> OverturnTrq/1
  vxtrans/1 -> Terminator1/1
  vytrans/1 -> Terminator2/1
  Rim_rotv/1 -> Terminator3/1
  InclinAngle/1 -> Terminator4/1
  muRoad/1 -> Terminator5/1
  Load/1 -> Terminator/1
  Ground1/1 -> Slp/1
  Ground6/1 -> LoadFrc/1
  Ground7/1 -> RollResist/1
  Ground8/1 -> AlignTrq/1

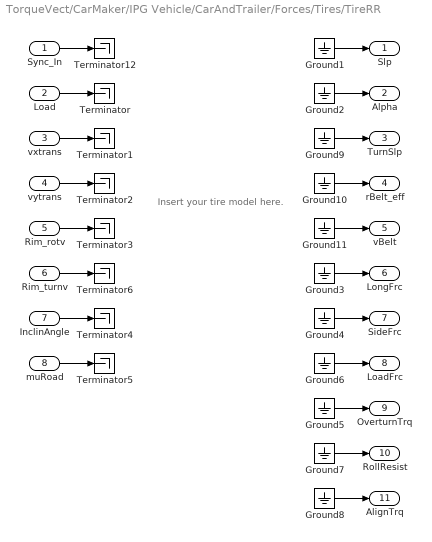
== system TorqueVect/CarMaker/IPG Vehicle/CarAndTrailer/Forces/Tires/TireRR ==
  note: Insert your tire model here.
  Sync_In : Inport
  Load : Inport  Port=2
  vxtrans : Inport  Port=3
  vytrans : Inport  Port=4
  Rim_rotv : Inport  Port=5
  Rim_turnv : Inport  Port=6
  InclinAngle : Inport  Port=7
  muRoad : Inport  Port=8
  Ground{1..11} (11 alike) : Ground
  Terminator{,1..6,12} (8 alike) : Terminator
  Slp : Outport
  Alpha : Outport  Port=2
  TurnSlp : Outport  Port=3
  rBelt_eff : Outport  Port=4
  vBelt : Outport  Port=5
  LongFrc : Outport  Port=6
  SideFrc : Outport  Port=7
  LoadFrc : Outport  Port=8
  OverturnTrq : Outport  Port=9
  RollResist : Outport  Port=10
  AlignTrq : Outport  Port=11
  wires:
  Ground11/1 -> vBelt/1
  Ground10/1 -> rBelt_eff/1
  Ground9/1 -> TurnSlp/1
  Rim_turnv/1 -> Terminator6/1
  Sync_In/1 -> Terminator12/1
  Ground2/1 -> Alpha/1
  Ground3/1 -> LongFrc/1
  Ground4/1 -> SideFrc/1
  Ground5/1 -> OverturnTrq/1
  vxtrans/1 -> Terminator1/1
  vytrans/1 -> Terminator2/1
  Rim_rotv/1 -> Terminator3/1
  InclinAngle/1 -> Terminator4/1
  muRoad/1 -> Terminator5/1
  Load/1 -> Terminator/1
  Ground1/1 -> Slp/1
  Ground6/1 -> LoadFrc/1
  Ground7/1 -> RollResist/1
  Ground8/1 -> AlignTrq/1

== system TorqueVect/CarMaker/IPG Vehicle/PowerTrain/PTControl Example/PTControl/PTC ==
  Constant2 : Constant
  Ground : Ground
  Mode_EngineDrive : Constant  Value=4
  Mux : Mux
  OperState_Driving : Constant  Value=4
  PTC MiscOut : Outport  VectorParamsAs1DForOutWhenUnconnected=off
  wires:
  Constant2/1 -> Mux/4  "Ignition"
  Mode_EngineDrive/1 -> Mux/3
  Ground/1 -> Mux/2  "OperationError"
  OperState_Driving/1 -> Mux/1
  Mux/1 -> PTC MiscOut/1

== system TorqueVect/CarMaker/IPG Vehicle/PowerTrain/PTControl Example/PTControl/Torque Control 0 ==
  note: Load_Motor0_FL
  note: Trq_trg
  Gas : Inport
  Add : Sum
  Constant2 : Constant  Value=TC_On
  Constant4 : Constant  Value=TV_On
  Electronic Gas Pedal FL : Subsystem
  Mux : Mux  Inputs=3
  NOTSET1 : Constant  Value=-99999
  NOTSET3 : Constant  Value=-99999
  Product1 : Product  RndMeth=Zero
  Scope : Scope
  Torque Vectoring FL : Subsystem
  MotorOut0 : Outport  VectorParamsAs1DForOutWhenUnconnected=off
  wires:
  Gas/1 -> Electronic Gas Pedal FL/2(VC.Gas)
  NOTSET1/1 -> Mux/3  "rotv_trg"
  NOTSET3/1 -> Mux/2
  Add/1 -> Scope/1, Mux/1
  Product1/1 -> Add/2
  Constant4/1 -> Product1/2
  Torque Vectoring FL/1(TV FL) -> Product1/1
  Electronic Gas Pedal FL/1(Motor_Gas_FL) -> Add/1
  Constant2/1 -> Electronic Gas Pedal FL/1(TV_On)
  Mux/1 -> MotorOut0/1

== system TorqueVect/CarMaker/IPG Vehicle/PowerTrain/PTControl Example/PTControl/Torque Control 1 ==
  note: Trq_trg
  note: Load_Motor1_FR
  Gas : Inport
  Add : Sum
  Constant2 : Constant  Value=TC_On
  Constant4 : Constant  Value=TV_On
  Electronic Gas Pedal FR : Subsystem
  Mux : Mux  Inputs=3
  NOTSET1 : Constant  Value=-99999
  NOTSET3 : Constant  Value=-99999
  Product1 : Product  RndMeth=Zero
  Torque Vectoring FR : Subsystem
  MotorOut1 : Outport  VectorParamsAs1DForOutWhenUnconnected=off
  wires:
  Gas/1 -> Electronic Gas Pedal FR/2(VC.Gas)
  Mux/1 -> MotorOut1/1
  Constant2/1 -> Electronic Gas Pedal FR/1(TV_On)
  Electronic Gas Pedal FR/1(Motor_Gas_FR) -> Add/1
  Torque Vectoring FR/1(TV FR) -> Product1/1
  Constant4/1 -> Product1/2
  Product1/1 -> Add/2
  Add/1 -> Mux/1
  NOTSET3/1 -> Mux/2
  NOTSET1/1 -> Mux/3  "rotv_trg"

== system TorqueVect/CarMaker/IPG Vehicle/PowerTrain/PTControl Example/PTControl/Torque Control 2 ==
  note: Trq_trg
  note: Load_Motor2_RL
  Gas : Inport
  Add : Sum
  Constant2 : Constant  Value=TC_On
  Constant4 : Constant  Value=TV_On
  Electronic Gas Pedal RL : Subsystem
  Mux : Mux  Inputs=3
  NOTSET1 : Constant  Value=-99999
  NOTSET3 : Constant  Value=-99999
  Product1 : Product  RndMeth=Zero
  Torque Vectoring RL : Subsystem
  MotorOut2 : Outport  VectorParamsAs1DForOutWhenUnconnected=off
  wires:
  Gas/1 -> Electronic Gas Pedal RL/2(VC.Gas)
  Mux/1 -> MotorOut2/1
  Constant2/1 -> Electronic Gas Pedal RL/1(TV_On)
  Electronic Gas Pedal RL/1(Motor_Gas_RL) -> Add/1
  Torque Vectoring RL/1(TV RL) -> Product1/1
  Constant4/1 -> Product1/2
  Product1/1 -> Add/2
  Add/1 -> Mux/1
  NOTSET3/1 -> Mux/2
  NOTSET1/1 -> Mux/3  "rotv_trg"

== system TorqueVect/CarMaker/IPG Vehicle/PowerTrain/PTControl Example/PTControl/Torque Control 3 ==
  note: Load_Motor3_RR
  note: Trq_trg
  Gas : Inport
  Add : Sum
  Constant2 : Constant  Value=TC_On
  Constant4 : Constant  Value=TV_On
  Electronic Gas Pedal RR : Subsystem
  Mux : Mux  Inputs=3
  NOTSET1 : Constant  Value=-99999
  NOTSET3 : Constant  Value=-99999
  Product1 : Product  RndMeth=Zero
  Torque Vectoring RR : Subsystem
  MotorOut3 : Outport  VectorParamsAs1DForOutWhenUnconnected=off
  wires:
  Gas/1 -> Electronic Gas Pedal RR/2(VC.Gas)
  NOTSET1/1 -> Mux/3  "rotv_trg"
  NOTSET3/1 -> Mux/2
  Add/1 -> Mux/1
  Product1/1 -> Add/2
  Constant4/1 -> Product1/2
  Torque Vectoring RR/1(TV RR) -> Product1/1
  Electronic Gas Pedal RR/1(Motor_Gas_RR) -> Add/1
  Constant2/1 -> Electronic Gas Pedal RR/1(TV_On)
  Mux/1 -> MotorOut3/1

== system TorqueVect/CarMaker/IPG Vehicle/PowerTrain/PTControl Example/PTControl_In/CreateBus PTC Battery ==
  In : Inport
  BusCreator : BusCreator  Inputs=14
  Demux : Demux  Outputs=14
      settings: DisplayOption=none
  Out : Outport  VectorParamsAs1DForOutWhenUnconnected=off
  wires:
  In/1 -> Demux/1
  BusCreator/1 -> Out/1
  Demux/1 -> BusCreator/1  "PTC BattLVIn SOC"
  Demux/2 -> BusCreator/2  "PTC BattLVIn SOH"
  Demux/3 -> BusCreator/3  "PTC BattLVIn Current"
  Demux/4 -> BusCreator/4  "PTC BattLVIn AOC"
  Demux/5 -> BusCreator/5  "PTC BattLVIn Temp"
  Demux/6 -> BusCreator/6  "PTC BattLVIn Energy"
  Demux/7 -> BusCreator/7  "PTC BattLVIn Pwr_max"
  Demux/8 -> BusCreator/8  "PTC BattHVIn SOC"
  Demux/9 -> BusCreator/9  "PTC BattHVIn SOH"
  Demux/10 -> BusCreator/10  "PTC BattHVIn Current"
  Demux/11 -> BusCreator/11  "PTC BattHVIn AOC"
  Demux/12 -> BusCreator/12  "PTC BattHVIn Temp"
  Demux/13 -> BusCreator/13  "PTC BattHVIn Energy"
  Demux/14 -> BusCreator/14  "PTC BattHVIn Pwr_max"

== system TorqueVect/CarMaker/IPG Vehicle/PowerTrain/PTControl Example/PTControl_In/CreateBus PTC ClutchIn ==
  In : Inport
  BusCreator : BusCreator  Inputs=6
  Demux : Demux  Outputs=6
      settings: DisplayOption=none
  Out : Outport  VectorParamsAs1DForOutWhenUnconnected=off
  wires:
  In/1 -> Demux/1
  BusCreator/1 -> Out/1
  Demux/1 -> BusCreator/1  "PTC ClutchIn Pos"
  Demux/2 -> BusCreator/2  "PTC ClutchIn rotv_in"
  Demux/3 -> BusCreator/3  "PTC ClutchIn rotv_out"
  Demux/4 -> BusCreator/4  "PTC ClutchIn Trq_in"
  Demux/5 -> BusCreator/5  "PTC ClutchIn Trq_out"
  Demux/6 -> BusCreator/6  "PTC ClutchIn i_TrqIn2Out"

== system TorqueVect/CarMaker/IPG Vehicle/PowerTrain/PTControl Example/PTControl_In/CreateBus PTC Control Units ==
  In : Inport
  BusCreator : BusCreator  Inputs=4
  Demux : Demux
      settings: DisplayOption=none
  Out : Outport  VectorParamsAs1DForOutWhenUnconnected=off
  wires:
  In/1 -> Demux/1
  BusCreator/1 -> Out/1
  Demux/1 -> BusCreator/1  "PTC ECU_Status"
  Demux/2 -> BusCreator/2  "PTC MCU_Status"
  Demux/3 -> BusCreator/3  "PTC TCU_Status"
  Demux/4 -> BusCreator/4  "PTC BCU_Status"

== system TorqueVect/CarMaker/IPG Vehicle/PowerTrain/PTControl Example/PTControl_In/CreateBus PTC DriveSrcIn ==
  In : Inport
  BusCreator : BusCreator  Inputs=4
  Demux : Demux
      settings: DisplayOption=none
  Out : Outport  VectorParamsAs1DForOutWhenUnconnected=off
  wires:
  In/1 -> Demux/1
  BusCreator/1 -> Out/1
  Demux/1 -> BusCreator/1  "PTC DriveSrcIn_d0 Trq_DriveSrc_trg"
  Demux/2 -> BusCreator/2  "PTC DriveSrcIn_d1 Trq_DriveSrc_trg"
  Demux/3 -> BusCreator/3  "PTC DriveSrcIn_d2 Trq_DriveSrc_trg"
  Demux/4 -> BusCreator/4  "PTC DriveSrcIn_d3 Trq_DriveSrc_trg"

== system TorqueVect/CarMaker/IPG Vehicle/PowerTrain/PTControl Example/PTControl_In/CreateBus PTC EngineIn ==
  In : Inport
  BusCreator : BusCreator  Inputs=7
  Demux : Demux  Outputs=7
      settings: DisplayOption=none
  Out : Outport  VectorParamsAs1DForOutWhenUnconnected=off
  wires:
  In/1 -> Demux/1
  BusCreator/1 -> Out/1
  Demux/1 -> BusCreator/1  "PTC EngineIn Engine_on"
  Demux/2 -> BusCreator/2  "PTC EngineIn rotv"
  Demux/3 -> BusCreator/3  "PTC EngineIn Trq"
  Demux/4 -> BusCreator/4  "PTC EngineIn TrqDrag"
  Demux/5 -> BusCreator/5  "PTC EngineIn TrqFull"
  Demux/6 -> BusCreator/6  "PTC EngineIn TrqOpt"
  Demux/7 -> BusCreator/7  "PTC EngineIn FuelFlow"

== system TorqueVect/CarMaker/IPG Vehicle/PowerTrain/PTControl Example/PTControl_In/CreateBus PTC GearBoxIn ==
  In : Inport
  BusCreator : BusCreator  Inputs=20
  Demux : Demux  Outputs=20
      settings: DisplayOption=none
  Out : Outport  VectorParamsAs1DForOutWhenUnconnected=off
  wires:
  In/1 -> Demux/1
  BusCreator/1 -> Out/1
  Demux/1 -> BusCreator/1  "PTC GearBoxIn GearNo"
  Demux/2 -> BusCreator/2  "PTC GearBoxIn GearNo_dis"
  Demux/3 -> BusCreator/3  "PTC GearBoxIn Trq_DriveSrc_trg"
  Demux/4 -> BusCreator/4  "PTC GearBoxIn i"
  Demux/5 -> BusCreator/5  "PTC GearBoxIn rotv_in"
  Demux/6 -> BusCreator/6  "PTC GearBoxIn rotv_out"
  Demux/7 -> BusCreator/7  "PTC GearBoxIn Trq_in"
  Demux/8 -> BusCreator/8  "PTC GearBoxIn Trq_out"
  Demux/9 -> BusCreator/9  "PTC GearBoxIn Clutch Pos"
  Demux/10 -> BusCreator/10  "PTC GearBoxIn Clutch rotv_in"
  Demux/11 -> BusCreator/11  "PTC GearBoxIn Clutch rotv_out"
  Demux/12 -> BusCreator/12  "PTC GearBoxIn Clutch Trq_in"
  Demux/13 -> BusCreator/13  "PTC GearBoxIn Clutch Trq_out"
  Demux/14 -> BusCreator/14  "PTC GearBoxIn Clutch i_TrqIn2Out"
  Demux/15 -> BusCreator/15  "PTC GearBoxIn Clutch_dis Pos"
  Demux/16 -> BusCreator/16  "PTC GearBoxIn Clutch_dis rotv_in"
  Demux/17 -> BusCreator/17  "PTC GearBoxIn Clutch_dis rotv_out"
  Demux/18 -> BusCreator/18  "PTC GearBoxIn Clutch_dis Trq_in"
  Demux/19 -> BusCreator/19  "PTC GearBoxIn Clutch_dis Trq_out"
  Demux/20 -> BusCreator/20  "PTC GearBoxIn Clutch_dis i_TrqIn2Out"

== system TorqueVect/CarMaker/IPG Vehicle/PowerTrain/PTControl Example/PTControl_In/CreateBus PTC GearBoxM_In0 ==
  In : Inport
  BusCreator : BusCreator  Inputs=20
  Demux : Demux  Outputs=20
      settings: DisplayOption=none
  Out : Outport  VectorParamsAs1DForOutWhenUnconnected=off
  wires:
  In/1 -> Demux/1
  BusCreator/1 -> Out/1
  Demux/1 -> BusCreator/1  "PTC GearBoxM_In0 GearNo"
  Demux/2 -> BusCreator/2  "PTC GearBoxM_In0 GearNo_dis"
  Demux/3 -> BusCreator/3  "PTC GearBoxM_In0 Trq_DriveSrc_trg"
  Demux/4 -> BusCreator/4  "PTC GearBoxM_In0 i"
  Demux/5 -> BusCreator/5  "PTC GearBoxM_In0 rotv_in"
  Demux/6 -> BusCreator/6  "PTC GearBoxM_In0 rotv_out"
  Demux/7 -> BusCreator/7  "PTC GearBoxM_In0 Trq_in"
  Demux/8 -> BusCreator/8  "PTC GearBoxM_In0 Trq_out"
  Demux/9 -> BusCreator/9  "PTC GearBoxM_In0 Clutch Pos"
  Demux/10 -> BusCreator/10  "PTC GearBoxM_In0 Clutch rotv_in"
  Demux/11 -> BusCreator/11  "PTC GearBoxM_In0 Clutch rotv_out"
  Demux/12 -> BusCreator/12  "PTC GearBoxM_In0 Clutch Trq_in"
  Demux/13 -> BusCreator/13  "PTC GearBoxM_In0 Clutch Trq_out"
  Demux/14 -> BusCreator/14  "PTC GearBoxM_In0 Clutch i_TrqIn2Out"
  Demux/15 -> BusCreator/15  "PTC GearBoxM_In0 Clutch_dis Pos"
  Demux/16 -> BusCreator/16  "PTC GearBoxM_In0 Clutch_dis rotv_in"
  Demux/17 -> BusCreator/17  "PTC GearBoxM_In0 Clutch_dis rotv_out"
  Demux/18 -> BusCreator/18  "PTC GearBoxM_In0 Clutch_dis Trq_in"
  Demux/19 -> BusCreator/19  "PTC GearBoxM_In0 Clutch_dis Trq_out"
  Demux/20 -> BusCreator/20  "PTC GearBoxM_In0 Clutch_dis i_TrqIn2Out"
